simulink model "beif"  (R2022a)
settings: Solver=FixedStepAuto  StartTime=0.0  StopTime=1.0  FixedStep=0.001  RelTol=1e-3
settings Model: Creator=Administrator  LastModifiedBy=Administrator

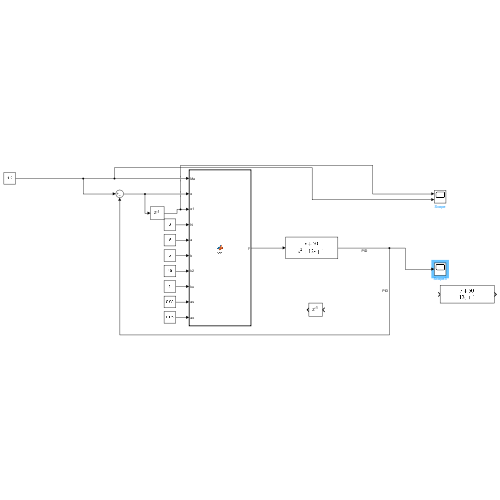
[thumbnail: Simulink's stored preview of the top-level diagram]
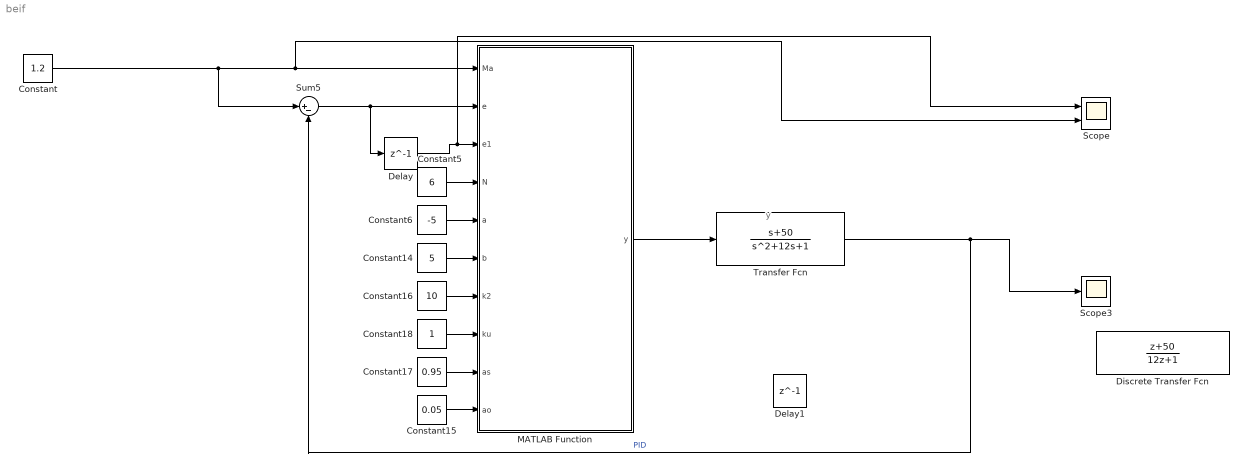
== system beif ==
  note: y
  Constant : Constant  Value=1.2
  Constant14 : Constant  Value=5  OutDataTypeStr=Inherit: Inherit via back propagation
  Constant15 : Constant  Value=0.05  OutDataTypeStr=Inherit: Inherit via back propagation
  Constant16 : Constant  Value=10  OutDataTypeStr=Inherit: Inherit via back propagation
  Constant17 : Constant  Value=0.95  OutDataTypeStr=Inherit: Inherit via back propagation
  Constant18 : Constant  OutDataTypeStr=Inherit: Inherit via back propagation
  Constant5 : Constant  Value=6  OutDataTypeStr=Inherit: Inherit via back propagation
  Constant6 : Constant  Value=-5
  Delay : Delay  DelayLength=1
  Delay1 : Delay  DelayLength=1  InitialCondition=0
  Discrete Transfer Fcn : DiscreteTransferFcn  Numerator=[1 50]  Denominator=[12 1]
  MATLAB Function : MATLAB Function  TreatAsAtomicUnit=on
      settings: MinAlgLoopOccurrences=on
  Scope : Scope  NumInputPorts=2
  Scope3 : Scope
  Sum5 : Sum  Inputs=|+-
  Transfer Fcn : TransferFcn  Numerator=[1 50]  Denominator=[1 12 1 ]
  wires:
  Constant6/1 -> MATLAB Function/5(a)
  Constant18/1 -> MATLAB Function/8(ku)
  Constant15/1 -> MATLAB Function/10(ao)
  Sum5/1 -> Delay/1, MATLAB Function/2(e)
  Constant5/1 -> MATLAB Function/4(N)
  Constant14/1 -> MATLAB Function/6(b)
  Constant16/1 -> MATLAB Function/7(k2)
  Constant17/1 -> MATLAB Function/9(as)
  Transfer Fcn/1 -> Sum5/2, Scope3/1  "PID"
  MATLAB Function/1(y) -> Transfer Fcn/1
  Constant/1 -> Scope/2, MATLAB Function/1(Ma), Sum5/1
  Delay/1 -> Scope/1, MATLAB Function/3(e1)

== matlab function beif/MATLAB Function ==
  data: Ma input; e input; e1 input; N input; y output; a input; b input; k2 input; ku input; as input; ao input
function y = fcn(Ma,e,e1,N,a,b,k2,ku,as,ao)


	ed = e - e1;
	E = -(2 * N) * (e * k2 - (a + b)) / (b - a);    
	E1 = E;
	EC = -(2 * N) * (ed - (a + b)) / (b - a);
	EC1 = 270 * EC;
	a1 = (1 / N) * (as - ao) * abs(E1) + ao;
	y1 = (-(a1 * E1 + (1 - a1) * EC1) / 2);
    y2=y1*ku;
    y=y2*Ma;
    
end
